simulink model "bank_tuner_tuner"  (R2022b)
settings: Solver=VariableStepAuto  StartTime=0.0  StopTime=20  RelTol=1e-3
undefined symbols (not defined in the file): CdProp, Ct, g, invControlMat, Ixx, Iyy, Izz, larm, mass
libraries: slpidlib x3, shared6dof x1
settings Model: Creator=aaron  LastModifiedBy=aaron

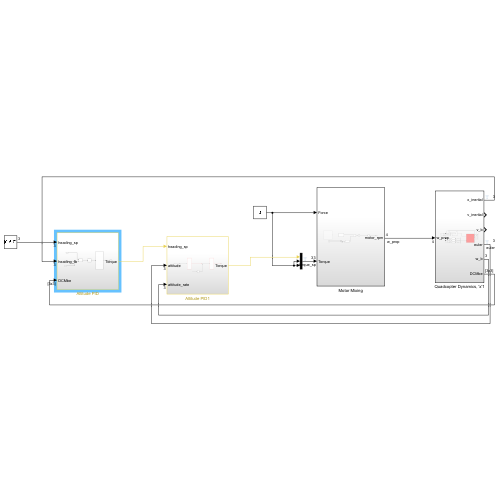
[thumbnail: Simulink's stored preview of the top-level diagram]
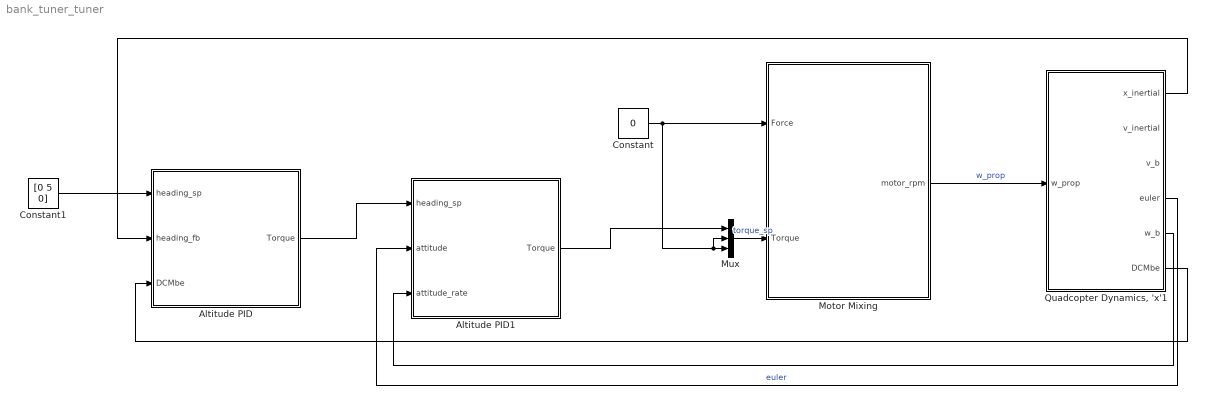
== system bank_tuner_tuner ==
  Altitude PID : Subsystem
  Altitude PID1 : Subsystem
  Constant : Constant  Value=0
  Constant1 : Constant  Value=[0 5 0]
  Motor Mixing : Subsystem
  Mux : Mux  Inputs=3
  "Quadcopter Dynamics, 'x'1" : Subsystem
  wires:
  Mux/1 -> Motor Mixing/2(Torque)  "torque_sp"
  Constant/1 -> Motor Mixing/1(Force), Mux/2, Mux/3
  Motor Mixing/1(motor_rpm) -> "Quadcopter Dynamics, 'x'1"/1(w_prop)  "w_prop"
  Constant1/1 -> Altitude PID/1(heading_sp)
  "Quadcopter Dynamics, 'x'1"/1(x_inertial) -> Altitude PID/2(heading_fb)
  "Quadcopter Dynamics, 'x'1"/6(DCMbe) -> Altitude PID/3(DCMbe)
  Altitude PID/1(Torque) -> Altitude PID1/1(heading_sp)
  "Quadcopter Dynamics, 'x'1"/4(euler) -> Altitude PID1/2(attitude)  "euler"
  "Quadcopter Dynamics, 'x'1"/5(w_b) -> Altitude PID1/3(attitude_rate)
  Altitude PID1/1(Torque) -> Mux/1

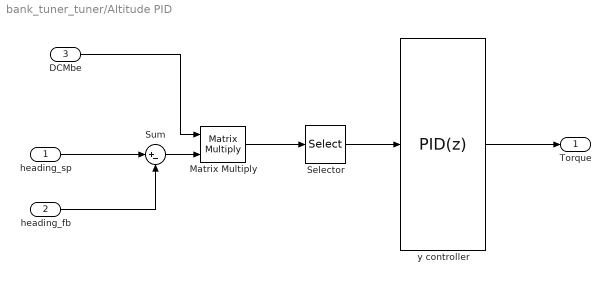
== system bank_tuner_tuner/Altitude PID ==
  heading_sp : Inport
  heading_fb : Inport  Port=2
  DCMbe : Inport  Port=3
  Matrix Multiply : Product  Multiplication=Matrix(*)
  Selector : Selector  InputPortWidth=3  IndexOptions=Index vector (dialog)  Indices=2  OutputSizes=1
  Sum : Sum  Inputs=|+-
  y controller : slpidlib/PID Controller  Controller=PID  Form=Parallel  TimeDomain=Discrete-time  UseExternalTs=off  SampleTime=-1  IntegratorMethod=Forward Euler  FilterMethod=Forward Euler  ControllerParametersSource=internal  P=0.0492870424099626  I=0.00562229643950214  UseKiTs=off  D=0.048634273252308  N=2.1798624918428  UseFilter=on  TunerSelectOption=Transfer Function Based (PID Tuner App)  InitialConditionSource=internal  InitialConditionForIntegrator=0  InitialConditionForFilter=0  DifferentiatorICPrevScaledInput=0  ExternalReset=none  TrackingMode=off  Kt=1  LimitOutput=off  SatLimitsSource=internal  UpperSaturationLimit=inf  LowerSaturationLimit=-inf  LinearizeAsGain=on  AntiWindupMode=clamping  Kb=1  LimitIntegrator=off  UpperIntegratorSaturationLimit=inf  LowerIntegratorSaturationLimit=-inf  POutMin=[]  POutMax=[]  IOutMin=[]  IOutMax=[]  DOutMin=[]  DOutMax=[]  NOutMin=[]  NOutMax=[]  SumOutMin=[]  SumOutMax=[]  SaturationOutMin=[]  SaturationOutMax=[]  PParamMin=[]  PParamMax=[]  IParamMin=[]  IParamMax=[]  DParamMin=[]  DParamMax=[]  NParamMin=[]  NParamMax=[]  KbParamMin=[]  KbParamMax=[]  KtParamMin=[]  KtParamMax=[]  KbOutMin=[]  KbOutMax=[]  KtOutMin=[]  KtOutMax=[]  IntegratorOutMin=[]  IntegratorOutMax=[]  FilterOutMin=[]  FilterOutMax=[]  SumI1OutMin=[]  SumI1OutMax=[]  SumI2OutMin=[]  SumI2OutMax=[]  SumI3OutMin=[]  SumI3OutMax=[]  SumI4OutMin=[]  SumI4OutMax=[]  SumDOutMin=[]  SumDOutMax=[]  DifferentiatorOutMin=[]  DifferentiatorOutMax=[]  FilterDiffOutCoefMin=[]  FilterDiffOutCoefMax=[]  ReciprocalOutMin=[]  ReciprocalOutMax=[]  SumDenOutMin=[]  SumDenOutMax=[]  SumNumOutMin=[]  SumNumOutMax=[]  DivideOutMin=[]  DivideOutMax=[]  UdiffTsProdOutMin=[]  UdiffTsProdOutMax=[]  NTsProdOutMin=[]  NTsProdOutMax=[]  UintegralTsProdOutMin=[]  UintegralTsProdOutMax=[]  UngainTsProdOutMin=[]  UngainTsProdOutMax=[]  ClampingZeroOutDataTypeStr=Inherit: Inherit via back propagation  ClampingZeroOutMin=[]  ClampingZeroOutMax=[]  FilterDenConstantOutDataTypeStr=Inherit: Inherit via back propagation  FilterDenConstantOutMin=[]  FilterDenConstantOutMax=[]  PCopyOutDataTypeStr=Inherit: Inherit via back propagation  PCopyOutMin=[]  PCopyOutMax=[]  NCopyOutDataTypeStr=Inherit: Inherit via back propagation  NCopyOutMin=[]  NCopyOutMax=[]  IntegratorContinuousStateAttributes=''  IntegratorStateMustResolveToSignalObject=off  IntegratorRTWStateStorageClass=Auto  FilterContinuousStateAttributes=''  FilterStateMustResolveToSignalObject=off  FilterRTWStateStorageClass=Auto  ParallelPVariant=InternalParameters  IdealPVariant=Disabled  IVariant=InternalParameters  DVariant=InternalParameters  IntegratorVariant=Discrete  SatVariant=Disabled  AWVariant=Passthrough  PCopyVariant=Disabled  TRVariant=Disabled  FdbkBlocksVariant=Forward  IdealPFdbkVariant=Disabled  SatFdbkVariant=Disabled  DerivativeFilterVariant=ForwardEulerFilter  NVariant=InternalParameters  NCopyVariant=Disabled  FilterICVariant=InternalICsFilter  IntegratorICVariant=InternalICs  ExternalResetVariant=Disabled  TRSumVariant=Passthrough  SumFdbkVariant=Disabled  SumVariant=Sum_PID  TsampFilterVariant=InternalTs  TsampNgainVariant=Passthrough  TsampIntegralVariant=Passthrough  ExternalSaturationOutDataTypeStr=Inherit: Same as second input
  Torque : Outport
  wires:
  Sum/1 -> Matrix Multiply/2
  heading_fb/1 -> Sum/2
  y controller/1 -> Torque/1
  heading_sp/1 -> Sum/1
  DCMbe/1 -> Matrix Multiply/1
  Matrix Multiply/1 -> Selector/1
  Selector/1 -> y controller/1

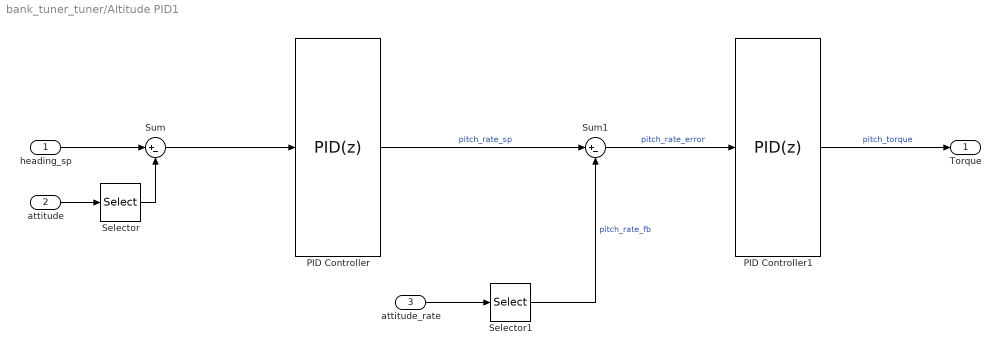
== system bank_tuner_tuner/Altitude PID1 ==
  heading_sp : Inport
  attitude : Inport  Port=2
  attitude_rate : Inport  Port=3
  PID Controller : slpidlib/PID Controller  Controller=PID  Form=Parallel  TimeDomain=Discrete-time  UseExternalTs=off  SampleTime=-1  IntegratorMethod=Forward Euler  FilterMethod=Forward Euler  ControllerParametersSource=internal  P=3.03667170880983  I=0.331567528847484  UseKiTs=off  D=0.829523975786847  N=4.93710017873255  UseFilter=on  TunerSelectOption=Transfer Function Based (PID Tuner App)  InitialConditionSource=internal  InitialConditionForIntegrator=0  InitialConditionForFilter=0  DifferentiatorICPrevScaledInput=0  ExternalReset=none  TrackingMode=off  Kt=1  LimitOutput=off  SatLimitsSource=internal  UpperSaturationLimit=inf  LowerSaturationLimit=-inf  LinearizeAsGain=on  AntiWindupMode=clamping  Kb=1  LimitIntegrator=off  UpperIntegratorSaturationLimit=inf  LowerIntegratorSaturationLimit=-inf  POutMin=[]  POutMax=[]  IOutMin=[]  IOutMax=[]  DOutMin=[]  DOutMax=[]  NOutMin=[]  NOutMax=[]  SumOutMin=[]  SumOutMax=[]  SaturationOutMin=[]  SaturationOutMax=[]  PParamMin=[]  PParamMax=[]  IParamMin=[]  IParamMax=[]  DParamMin=[]  DParamMax=[]  NParamMin=[]  NParamMax=[]  KbParamMin=[]  KbParamMax=[]  KtParamMin=[]  KtParamMax=[]  KbOutMin=[]  KbOutMax=[]  KtOutMin=[]  KtOutMax=[]  IntegratorOutMin=[]  IntegratorOutMax=[]  FilterOutMin=[]  FilterOutMax=[]  SumI1OutMin=[]  SumI1OutMax=[]  SumI2OutMin=[]  SumI2OutMax=[]  SumI3OutMin=[]  SumI3OutMax=[]  SumI4OutMin=[]  SumI4OutMax=[]  SumDOutMin=[]  SumDOutMax=[]  DifferentiatorOutMin=[]  DifferentiatorOutMax=[]  FilterDiffOutCoefMin=[]  FilterDiffOutCoefMax=[]  ReciprocalOutMin=[]  ReciprocalOutMax=[]  SumDenOutMin=[]  SumDenOutMax=[]  SumNumOutMin=[]  SumNumOutMax=[]  DivideOutMin=[]  DivideOutMax=[]  UdiffTsProdOutMin=[]  UdiffTsProdOutMax=[]  NTsProdOutMin=[]  NTsProdOutMax=[]  UintegralTsProdOutMin=[]  UintegralTsProdOutMax=[]  UngainTsProdOutMin=[]  UngainTsProdOutMax=[]  ClampingZeroOutDataTypeStr=Inherit: Inherit via back propagation  ClampingZeroOutMin=[]  ClampingZeroOutMax=[]  FilterDenConstantOutDataTypeStr=Inherit: Inherit via back propagation  FilterDenConstantOutMin=[]  FilterDenConstantOutMax=[]  PCopyOutDataTypeStr=Inherit: Inherit via back propagation  PCopyOutMin=[]  PCopyOutMax=[]  NCopyOutDataTypeStr=Inherit: Inherit via back propagation  NCopyOutMin=[]  NCopyOutMax=[]  IntegratorContinuousStateAttributes=''  IntegratorStateMustResolveToSignalObject=off  IntegratorRTWStateStorageClass=Auto  FilterContinuousStateAttributes=''  FilterStateMustResolveToSignalObject=off  FilterRTWStateStorageClass=Auto  ParallelPVariant=InternalParameters  IdealPVariant=Disabled  IVariant=InternalParameters  DVariant=InternalParameters  IntegratorVariant=Discrete  SatVariant=Disabled  AWVariant=Passthrough  PCopyVariant=Disabled  TRVariant=Disabled  FdbkBlocksVariant=Forward  IdealPFdbkVariant=Disabled  SatFdbkVariant=Disabled  DerivativeFilterVariant=ForwardEulerFilter  NVariant=InternalParameters  NCopyVariant=Disabled  FilterICVariant=InternalICsFilter  IntegratorICVariant=InternalICs  ExternalResetVariant=Disabled  TRSumVariant=Passthrough  SumFdbkVariant=Disabled  SumVariant=Sum_PID  TsampFilterVariant=InternalTs  TsampNgainVariant=Passthrough  TsampIntegralVariant=Passthrough  ExternalSaturationOutDataTypeStr=Inherit: Same as second input
  PID Controller1 : slpidlib/PID Controller  Controller=PID  Form=Parallel  TimeDomain=Discrete-time  UseExternalTs=off  SampleTime=-1  IntegratorMethod=Forward Euler  FilterMethod=Forward Euler  ControllerParametersSource=internal  P=0.0206583329852232  I=0.0039692862708644  UseKiTs=off  D=-8.29964743746167e-05  N=4.89768405798445  UseFilter=on  TunerSelectOption=Transfer Function Based (PID Tuner App)  InitialConditionSource=internal  InitialConditionForIntegrator=0  InitialConditionForFilter=0  DifferentiatorICPrevScaledInput=0  ExternalReset=none  TrackingMode=off  Kt=1  LimitOutput=off  SatLimitsSource=internal  UpperSaturationLimit=inf  LowerSaturationLimit=-inf  LinearizeAsGain=on  AntiWindupMode=clamping  Kb=1  LimitIntegrator=off  UpperIntegratorSaturationLimit=inf  LowerIntegratorSaturationLimit=-inf  POutMin=[]  POutMax=[]  IOutMin=[]  IOutMax=[]  DOutMin=[]  DOutMax=[]  NOutMin=[]  NOutMax=[]  SumOutMin=[]  SumOutMax=[]  SaturationOutMin=[]  SaturationOutMax=[]  PParamMin=[]  PParamMax=[]  IParamMin=[]  IParamMax=[]  DParamMin=[]  DParamMax=[]  NParamMin=[]  NParamMax=[]  KbParamMin=[]  KbParamMax=[]  KtParamMin=[]  KtParamMax=[]  KbOutMin=[]  KbOutMax=[]  KtOutMin=[]  KtOutMax=[]  IntegratorOutMin=[]  IntegratorOutMax=[]  FilterOutMin=[]  FilterOutMax=[]  SumI1OutMin=[]  SumI1OutMax=[]  SumI2OutMin=[]  SumI2OutMax=[]  SumI3OutMin=[]  SumI3OutMax=[]  SumI4OutMin=[]  SumI4OutMax=[]  SumDOutMin=[]  SumDOutMax=[]  DifferentiatorOutMin=[]  DifferentiatorOutMax=[]  FilterDiffOutCoefMin=[]  FilterDiffOutCoefMax=[]  ReciprocalOutMin=[]  ReciprocalOutMax=[]  SumDenOutMin=[]  SumDenOutMax=[]  SumNumOutMin=[]  SumNumOutMax=[]  DivideOutMin=[]  DivideOutMax=[]  UdiffTsProdOutMin=[]  UdiffTsProdOutMax=[]  NTsProdOutMin=[]  NTsProdOutMax=[]  UintegralTsProdOutMin=[]  UintegralTsProdOutMax=[]  UngainTsProdOutMin=[]  UngainTsProdOutMax=[]  ClampingZeroOutDataTypeStr=Inherit: Inherit via back propagation  ClampingZeroOutMin=[]  ClampingZeroOutMax=[]  FilterDenConstantOutDataTypeStr=Inherit: Inherit via back propagation  FilterDenConstantOutMin=[]  FilterDenConstantOutMax=[]  PCopyOutDataTypeStr=Inherit: Inherit via back propagation  PCopyOutMin=[]  PCopyOutMax=[]  NCopyOutDataTypeStr=Inherit: Inherit via back propagation  NCopyOutMin=[]  NCopyOutMax=[]  IntegratorContinuousStateAttributes=''  IntegratorStateMustResolveToSignalObject=off  IntegratorRTWStateStorageClass=Auto  FilterContinuousStateAttributes=''  FilterStateMustResolveToSignalObject=off  FilterRTWStateStorageClass=Auto  ParallelPVariant=InternalParameters  IdealPVariant=Disabled  IVariant=InternalParameters  DVariant=InternalParameters  IntegratorVariant=Discrete  SatVariant=Disabled  AWVariant=Passthrough  PCopyVariant=Disabled  TRVariant=Disabled  FdbkBlocksVariant=Forward  IdealPFdbkVariant=Disabled  SatFdbkVariant=Disabled  DerivativeFilterVariant=ForwardEulerFilter  NVariant=InternalParameters  NCopyVariant=Disabled  FilterICVariant=InternalICsFilter  IntegratorICVariant=InternalICs  ExternalResetVariant=Disabled  TRSumVariant=Passthrough  SumFdbkVariant=Disabled  SumVariant=Sum_PID  TsampFilterVariant=InternalTs  TsampNgainVariant=Passthrough  TsampIntegralVariant=Passthrough  ExternalSaturationOutDataTypeStr=Inherit: Same as second input
  Selector : Selector  InputPortWidth=3  IndexOptions=Index vector (dialog)  Indices=1  OutputSizes=1
  Selector1 : Selector  InputPortWidth=3  IndexOptions=Index vector (dialog)  Indices=1  OutputSizes=1
  Sum : Sum  Inputs=|+-
  Sum1 : Sum  Inputs=|+-
  Torque : Outport
  wires:
  attitude/1 -> Selector/1
  Sum/1 -> PID Controller/1
  PID Controller1/1 -> Torque/1  "pitch_torque"
  Selector/1 -> Sum/2
  attitude_rate/1 -> Selector1/1
  Selector1/1 -> Sum1/2  "pitch_rate_fb"
  Sum1/1 -> PID Controller1/1  "pitch_rate_error"
  PID Controller/1 -> Sum1/1  "pitch_rate_sp"
  heading_sp/1 -> Sum/1

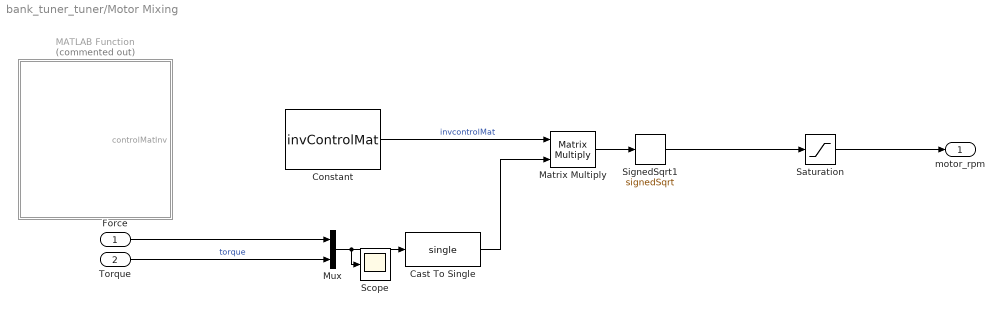
== system bank_tuner_tuner/Motor Mixing ==
  Force : Inport
  Torque : Inport  Port=2
  Cast To Single : DataTypeConversion  OutDataTypeStr=single  SaturateOnIntegerOverflow=off  RndMeth=Floor
  Constant : Constant  Value=invControlMat
  MATLAB Function : MATLAB Function  Commented=on  TreatAsAtomicUnit=on
  Matrix Multiply : Product  Multiplication=Matrix(*)
  Mux : Mux  Inputs=2
  Saturation : Saturate  UpperLimit=2000  LowerLimit=0
  Scope : Scope
  SignedSqrt1 : Sqrt  Operator=signedSqrt  IntermediateResultsDataTypeStr=single
  motor_rpm : Outport
  wires:
  Torque/1 -> Mux/2  "torque"
  Force/1 -> Mux/1
  Saturation/1 -> motor_rpm/1
  SignedSqrt1/1 -> Saturation/1
  Matrix Multiply/1 -> SignedSqrt1/1
  Constant/1 -> Matrix Multiply/1  "invcontrolMat"
  Cast To Single/1 -> Matrix Multiply/2
  Mux/1 -> Scope/1, Cast To Single/1

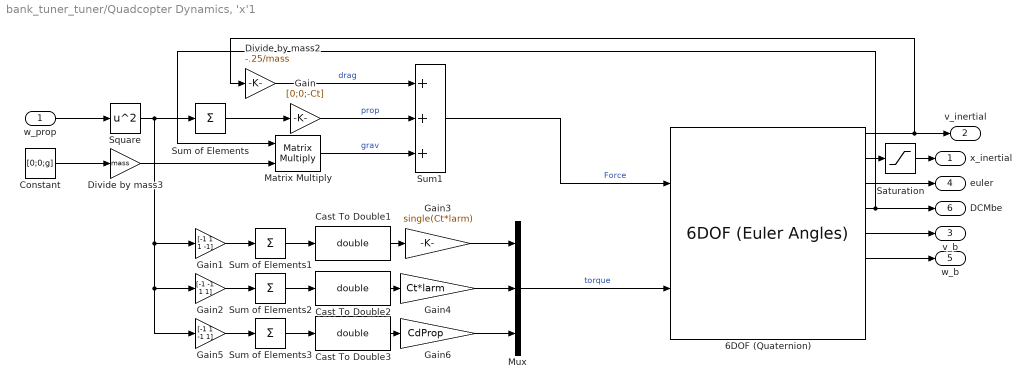
== system bank_tuner_tuner/Quadcopter Dynamics, 'x'1 ==
  w_prop : Inport
  6DOF (Quaternion) : shared6dof/6DOF (Euler Angles)  units=Metric (MKS)  mtype=Fixed  rep=Euler Angles  xme_0=[0,0,0]  Vm_0=[0,0,0]  eul_0=[0,0,0]  pm_0=[0,0,0]  mass_0=mass  mass_e=0.5  mass_f=2.0  inertia=diag([Ixx Iyy Izz])  inertia_e=eye(3)  inertia_f=2*eye(3)  k_quat=Vehicle.SixDOF.quatGain  vre_flag=on  abi_flag=on  aMode=aMode  xme_statename=''  Vm_statename=''  eul_statename=''  quat_statename=''  pm_statename=''  mass_statename=''
  Cast To Double1 : DataTypeConversion  OutDataTypeStr=double  SaturateOnIntegerOverflow=off  RndMeth=Floor
  Cast To Double2 : DataTypeConversion  OutDataTypeStr=double  SaturateOnIntegerOverflow=off  RndMeth=Floor
  Cast To Double3 : DataTypeConversion  OutDataTypeStr=double  SaturateOnIntegerOverflow=off  RndMeth=Floor
  Constant : Constant  Value=[0;0;g]
  Divide by mass2 : Gain  Gain=-.25/mass
  Divide by mass3 : Gain  Gain=mass
  Gain : Gain  Gain=[0;0;-Ct]
  Gain1 : Gain  Gain=[-1 1 1 -1]
  Gain2 : Gain  Gain=[-1 -1 1 1]
  Gain3 : Gain  Gain=single(Ct*larm)
  Gain4 : Gain  Gain=Ct*larm
  Gain5 : Gain  Gain=[-1 1 -1 1]
  Gain6 : Gain  Gain=CdProp
  Matrix Multiply : Product  Multiplication=Matrix(*)
  Mux : Mux  Inputs=3
  Saturation : Saturate  UpperLimit=[inf inf 0]  LowerLimit=-inf
  Square : Math  Operator=square
  Sum of Elements{,1..3} (4 alike) : Sum  Inputs=+
  Sum1 : Sum  Inputs=+++
  x_inertial : Outport
  v_inertial : Outport  Port=2
  v_b : Outport  Port=3
  euler : Outport  Port=4
  w_b : Outport  Port=5
  DCMbe : Outport  Port=6
  wires:
  Sum1/1 -> 6DOF (Quaternion)/1  "Force"
  Constant/1 -> Divide by mass3/1
  6DOF (Quaternion)/1 -> v_inertial/1, Divide by mass2/1
  Divide by mass2/1 -> Sum1/1  "drag"
  w_prop/1 -> Square/1
  Square/1 -> Gain5/1, Gain2/1, Gain1/1, Sum of Elements/1
  Sum of Elements/1 -> Gain/1
  Gain/1 -> Sum1/2  "prop"
  Gain1/1 -> Sum of Elements1/1
  Gain2/1 -> Sum of Elements2/1
  Gain5/1 -> Sum of Elements3/1
  Gain3/1 -> Mux/1
  Gain4/1 -> Mux/2
  Gain6/1 -> Mux/3
  Mux/1 -> 6DOF (Quaternion)/2  "torque"
  6DOF (Quaternion)/5 -> v_b/1
  6DOF (Quaternion)/2 -> Saturation/1
  6DOF (Quaternion)/6 -> w_b/1
  6DOF (Quaternion)/3 -> euler/1
  6DOF (Quaternion)/4 -> Matrix Multiply/1, DCMbe/1
  Cast To Double1/1 -> Gain3/1
  Sum of Elements1/1 -> Cast To Double1/1
  Cast To Double2/1 -> Gain4/1
  Sum of Elements2/1 -> Cast To Double2/1
  Sum of Elements3/1 -> Cast To Double3/1
  Cast To Double3/1 -> Gain6/1
  Saturation/1 -> x_inertial/1
  Divide by mass3/1 -> Matrix Multiply/2
  Matrix Multiply/1 -> Sum1/3  "grav"

== matlab function bank_tuner_tuner/Motor Mixing/MATLAB Function ==
  data: controlMatInv output; Ct parameter; larm parameter; CdProp parameter
function controlMatInv = calc_motor_speed(Ct,...
larm, CdProp)
% u1 = force;
% u2 = torques(1);
% u3 = torques(2);
% u4 = torques(3);


K = Ct;
L = larm;
C = CdProp;

% invControlMat = -[(C*u2 + C*u3 + C*L*u1 + K*L*u4)/(4*C*K*L);
%  (C*u2 - C*u3 - C*L*u1 + K*L*u4)/(4*C*K*L);
%  (C*u2 + C*u3 - C*L*u1 - K*L*u4)/(4*C*K*L);
% -(C*u2 - C*u3 + C*L*u1 - K*L*u4)/(4*C*K*L)];

invControlMat = [-1/(4*K), -1/(4*K*L), -1/(4*K*L), -1/(4*C);
                -1/(4*K),  1/(4*K*L), -1/(4*K*L),  1/(4*C);
                -1/(4*K),  1/(4*K*L),  1/(4*K*L), -1/(4*C);
                -1/(4*K), -1/(4*K*L),  1/(4*K*L),  1/(4*C)];
controlMatInv = invControlMat;
